simulink model "Eq_Euler_fcn_block"  (R2018a)
settings: Solver=VariableStepAuto  StartTime=0.0  StopTime=10.0  RelTol=1e-3
settings Model: Creator=LabT5  LastModifiedBy=LabT5

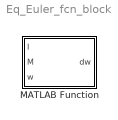
== system Eq_Euler_fcn_block ==
  MATLAB Function : MATLAB Function  TreatAsAtomicUnit=on

== matlab function Eq_Euler_fcn_block/MATLAB Function ==
  data: I input; dw output; M input; w input
function dw = Eq_Euler(I,M,w)
wx = w(1);
wy = w(2);
wz = w(3);
Ix = I(1);
Iy = I(2);
Iz = I(3);

Mx = M(1);
My = M(2);
Mz = M(3);

dwx = (Mx - wy*wz*(Iz - Iy))/Ix;
dwy = (My - wx*wz*(Ix - Iz))/Iy;
dwz = (Mz - wx*wy*(Iy - Ix))/Iz;

dw=[dwx dwy dwz]';
